simulink model "motor_brb"  (R2025a)
settings: Solver=FixedStepAuto  StartTime=0  StopTime=5  FixedStep=1e-4  RelTol=1e-3
undefined symbols (not defined in the file): f_supply, fault_severity, Torque_in, V_in
libraries: spsAsynchronousMachineSIUnitsLib x1, spsThreePhaseSourceLib x1, sps_lib x1
settings Model: Creator=User  LastModifiedBy=User
settings DataIOCC: SaveOutput=off  DSMLogging=off  ReturnWorkspaceOutputs=off

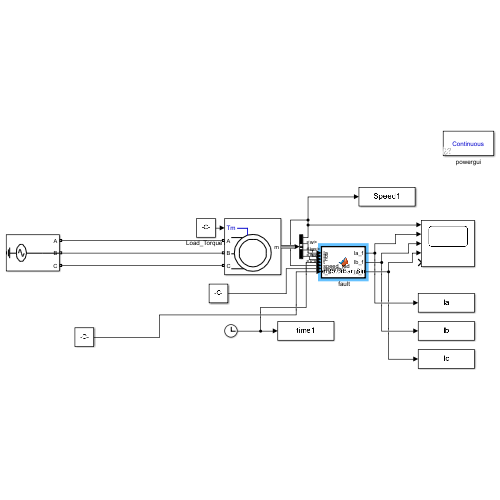
[thumbnail: Simulink's stored preview of the top-level diagram]
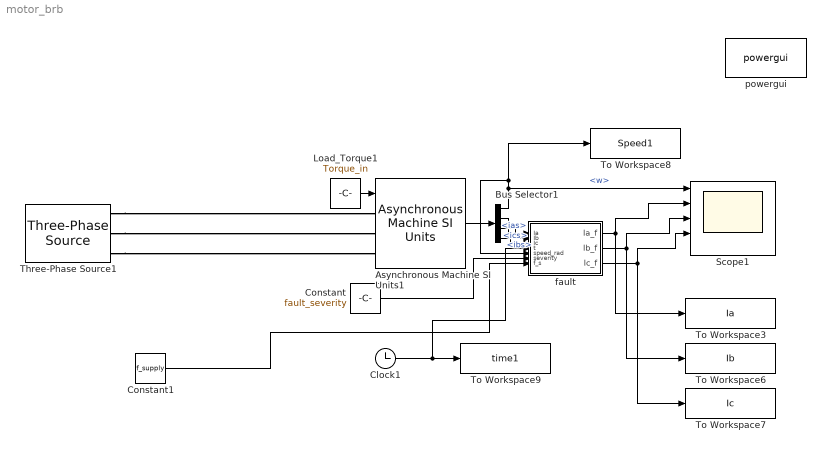
== system motor_brb ==
  " fault" : MATLAB Function  TreatAsAtomicUnit=on
  Asynchronous Machine SI Units1 : spsAsynchronousMachineSIUnitsLib/Asynchronous Machine SI Units  RotorType=Squirrel-cage  PresetModel=No  MechanicalLoad=Torque Tm  ShowDetailedParameters=on  ReferenceFrame=Stationary  Units=SI  MeasurementBus=on  NominalParameters=[7500 400 50]  VoltageRatio=1  Stator=[1.405 0.005839]  Rotor=[2 0.006839]  Cage1=[0.4155 0.002066]  Cage2=[0.4168 0.0003495]  Lm=0.1722  Mechanical=[0.0131 0.001 2]  PolePairs=2  InitialConditions=[0 0 0 0 0 0 0 0]  SimulateSaturation=off  Saturation=[14.03593122, 27.81365428, 53.79336849, 72.68890987, 97.98006896, 148.6815601, 215.7428561, 302.9841135, 428.7778367 ; 230, 322, 414, 460, 506, 552, 598, 644, 690]  LoadFlowParameters=1492000  TsPowergui=0  TsBlock=-1  IterativeModel=Trapezoidal non iterative  IterativeDiscreteModel=Trapezoidal non iterative  Pmec=1.492e+006
  Bus Selector1 : BusSelector  OutputSignals=w,ias,ibs,ics
  Clock1 : Clock
  Constant : Constant  Value=fault_severity
  Constant1 : Constant  Value=f_supply
  Load_Torque1 : Constant  Value=Torque_in
  Scope1 : Scope  NumInputPorts=5
      settings: ActiveDisplayYMinimum=-0.10260402762324485  ActiveDisplayYMaximum=0.098015223239877339
  Three-Phase Source1 : spsThreePhaseSourceLib/Three-Phase Source  InternalConnection=Yg  VoltagePhases=on  Voltage=400  PhaseAngle=0  Voltage_phases=[V_in V_in V_in]/sqrt(3)  PhaseAngles_phases=[0 -120 +120]  Frequency=f_supply  NonIdealSource=off  SpecifyImpedance=off  Resistance=0.8929  Inductance=16.58e-3  ShortCircuitLevel=100e6  BaseVoltage=25e3  XRratio=7  BusType=swing  Pref=10e3  Qref=0  Prefabc=[10e3, 10e3, 10e3]  Qrefabc=[0, 0, 0]  Qmin=-inf  Qmax=inf
  To Workspace3 : ToWorkspace  VariableName=Ia  SampleTime=-1
  To Workspace6 : ToWorkspace  VariableName=Ib  SampleTime=-1
  To Workspace7 : ToWorkspace  VariableName=Ic  SampleTime=-1
  To Workspace8 : ToWorkspace  VariableName=Speed1  SampleTime=-1
  To Workspace9 : ToWorkspace  VariableName=time1  SampleTime=-1
  powergui : sps_lib/powergui  Priority=1  SimulationMode=Continuous  SampleTime=50e-6  frequency=60  Iterations=50  frequencyindice=50  Pbase=100e6  ErrMax=1e-4  UnitsV=kV  UnitsW=MW  buscounter=0  FunctionMessages=off  echomessages=off  EnableUseOfTLC=off  CurrentSourceSwitches=off  DisableSnubberDevices=off  DisableRonSwitches=off  DisableVfSwitches=off  DisplayEquations=off  AutomaticDiscreteSolvers=off  SolverType=Tustin/Backward Euler (TBE)  Interpol=off  ExternalGateDelay=off  methode=off  Ts=100  x0status=blocks  SPID=on  SwTol=0  HookPort=off  NonlinearTolerance=1e-4  nMaxIteration=100  ContinueOnMaxIteration=off  RestoreLinks=warning  ResistiveCurrentMeasurement=off  Frange=[0:2:500]  Ylog=off  Xlog=on  ShowGrid=off  save=off  variable=ZData  structure=0  ZoomFFT=off  StartTime=0.0  cycles=1  DisplayStyle=1  fundamental=60  FreqAxis=off  MaxFrequency=1000  frequencyindicesteady=1  RmsSteady=1  display=off
  wires:
  Clock1/1 -> " fault"/4(t), To Workspace9/1
  Asynchronous Machine SI Units1/1 -> Bus Selector1/1
  Bus Selector1/1 -> Scope1/1, To Workspace8/1, " fault"/5(speed_rad)  "<w>"
  Load_Torque1/1 -> Asynchronous Machine SI Units1/1
  " fault"/1(Ia_f) -> Scope1/2, To Workspace3/1
  " fault"/2(Ib_f) -> Scope1/3, To Workspace6/1
  " fault"/3(Ic_f) -> Scope1/4, To Workspace7/1
  Bus Selector1/2 -> " fault"/1(Ia)  "<ias>"
  Bus Selector1/3 -> " fault"/2(Ib)  "<ibs>"
  Bus Selector1/4 -> " fault"/3(Ic)  "<ics>"
  Constant/1 -> " fault"/6(severity)
  Constant1/1 -> " fault"/7(f_s)
  connections:
  Three-Phase Source1/RConn2 -- Asynchronous Machine SI Units1/LConn2
  Three-Phase Source1/RConn1 -- Asynchronous Machine SI Units1/LConn1
  Three-Phase Source1/RConn3 -- Asynchronous Machine SI Units1/LConn3

== matlab function motor_brb/ fault ==
  data: Ia input; Ia_f output; Ib input; Ic input; t input; Ib_f output; Ic_f output; speed_rad input; severity input; f_s input
function [Ia_f, Ib_f, Ic_f] = BrokenRotorBar_Simulink(Ia, Ib, Ic, t, speed_rad, severity, f_s)
    %#codegen
    % CORRECTED BROKEN ROTOR BAR FAULT MODEL
    % Physics: Amplitude Modulation (AM) of Stator Current
    
    % --- 1. Motor Parameters ---

    sync_speed = 120 *(f_s / 4);    % For 4-pole / 50Hz
    speed_rpm = speed_rad * 9.549;
    % Ensure speed is scalar if passed as vector (taking mean or first element)
    if ~isscalar(speed_rpm)
        current_speed = speed_rpm(1); 
    else
        current_speed = speed_rpm;
    end

    % --- 2. Calculate Slip & Fault Frequency ---
    % Slip s = (Ns - Nr) / Ns
    s = (sync_speed - current_speed) / sync_speed;
    
    % Clamp slip to realistic positive values (avoid division by zero or negative slip)
    if s < 0.001, s = 0.001; end
    
    % Modulation Frequency = 2 * s * fs (Characteristic BRB Frequency)
    f_brb = 2.0 * s * f_s; 
    
    % --- 3. Modulation Depth (THE FIX) ---
    % Realism adjustment:
    % Severity 1.0 should roughly equal 5-10% sideband amplitude.
    % Since Sideband Amp = m/2, we need m = 0.10 to 0.20.
    
    % Let's set Max Modulation (m) = 0.15 (15%) for severity=1.
    % This results in sidebands of 7.5%, which is a very strong fault pattern.
    modulation_depth = severity * 0.10; 
    
    % --- 4. Apply Modulation ---
    if severity > 0
        % Phase A Modulation (0 deg)
        mod_a = 1 + modulation_depth * cos(2*pi*f_brb*t);
        
        % Phase B Modulation (-120 deg shift relative to A)
        % The fault rotates, so the envelope arrives at Phase B later.
        mod_b = 1 + modulation_depth * cos(2*pi*f_brb*t - 2*pi/3);
        
        % Phase C Modulation (+120 deg shift relative to A)
        mod_c = 1 + modulation_depth * cos(2*pi*f_brb*t + 2*pi/3);
        
        Ia_f = Ia .* mod_a;
        Ib_f = Ib .* mod_b;
        Ic_f = Ic .* mod_c;
        

    else
        % Healthy State
        Ia_f = Ia; 
        Ib_f = Ib; 
        Ic_f = Ic;
    end
end
